simulink subsystem "battery_96_pack"  (R2022b)
settings: Solver=VariableStepAuto  StartTime=0.0  StopTime=10.0  RelTol=1e-3
values from neighbouring files (symbols this model uses):
  initial_temperature = 288.15    [battery_pack_model_data.sldd]
libraries: fl_lib x3, nesl_utility x1
settings Model: Creator=tshintai  LastModifiedBy=tshintai
settings ModelReferenceCC: EnableRefExpFcnMdlSchedulingChecks=on

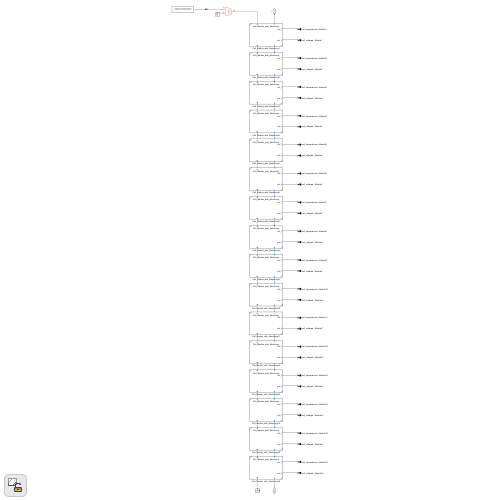
[thumbnail: Simulink's stored preview of the top-level diagram]
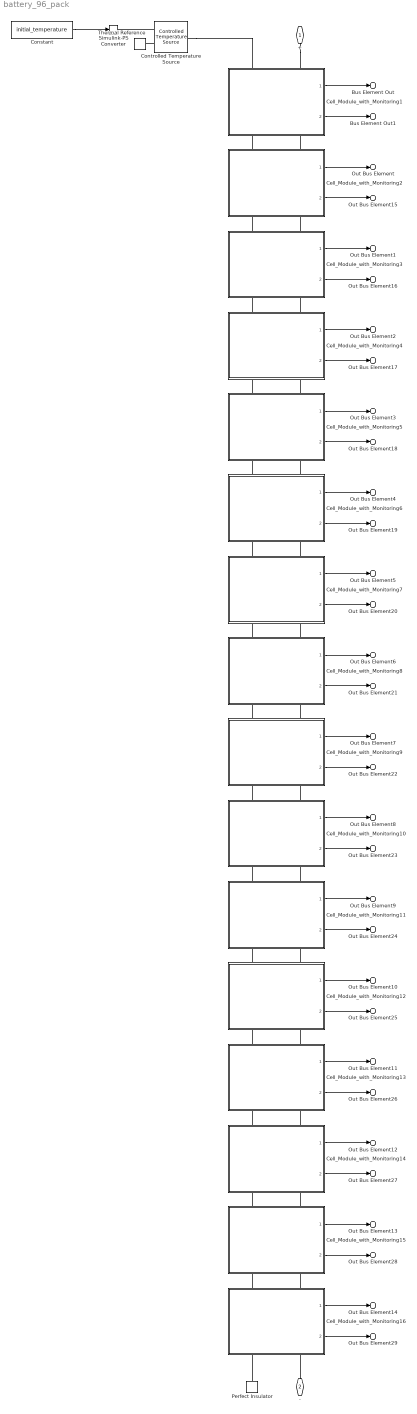
== system battery_96_pack ==
  Cell_Module_with_Monitoring{1..16} (16 alike) : Subsystem  ReferencedSubsystem=Cell_Module_with_Monitoring
      settings: PortSchema="{\"entries\":[{\"content\":{\"sides\":[{\"content\":{\"connectorIds\":[]},\"type\":\"ConnectorPlacement.EquallySpacedRectSide\",\"uuid\":\"dcef24a5-8142-4849-86b9-b18f022ccde6\"},{\"content\":{\"connectorIds\":[\"Out1\",\"Out2\"],\"side\":\"RIGHT\"},\"type\":\"ConnectorPlacement.EquallySpacedRectSide\",\"uuid\":\"d6f70724-8f5a-4fbe-99a3-1d7744c6c20b\"},{\"content\":{\"connectorIds\":[\"LConn2\",\"LConn1\"],\"side\":\"TOP\"},\"type\":\"ConnectorPlacement.EquallySpacedRectSide\",\"uuid\":\"1a464afb-99ff-42a4-8ba4-5eff5af9414c\"},{\"content\":{\"connectorIds\":[\"RConn2\",\"RConn1\"],\"side\":\"BOTTOM\"},\"type\":\"ConnectorPlacement.EquallySpacedRectSide\",\"uuid\":\"74a9329d-ffaf-4bfc-bec3-31f00c72c9b7\"}]},\"type\":\"ConnectorPlacement.EquallySpacedConnector\",\"uuid\":\"3b26f8a7-d97e-4bd5-81c6-74f00c6fb23d\"}],\"packageUris\":[\"http://schema.mathworks.com/mf0/Connector/R2020b\"],\"version\":\"1.0\"}"
  Constant : Constant  Value=initial_temperature
  Controlled Temperature Source : fl_lib/Thermal/Thermal Sources/Controlled Temperature Source
  Perfect Insulator : fl_lib/Thermal/Thermal Elements/Perfect Insulator  T_specify=off  T_priority=None  T=0 K  T_nominal_specify=off  T_nominal_unit=K  T_nominal_value=1
  Simulink-PS Converter : nesl_utility/Simulink-PS Converter  PhysicalDomain=network_engine_domain  SubClassName=ps_input  LeftPortType=input  RightPortType=output  PseudoPeriodic=off  Frequencies=[]  NoiseDistribution=none  NoiseParameters=[]  Unit=K  AffineConversion=on  FilteringAndDerivatives=provide  SimscapeFilterOrder=1  InputFilterTimeConstant=0.001  UdotUserProvided=0
  Thermal Reference : fl_lib/Thermal/Thermal Elements/Thermal Reference
  + : PMIOPort  Side=Left
  - : PMIOPort  Port=2  Side=Right
  Bus Element Out : Outport  PortName=cell_temperatures  Element=Module1
  Out Bus Element : Outport  PortName=cell_temperatures  Element=Module2
  Out Bus Element1 : Outport  PortName=cell_temperatures  Element=Module3
  Out Bus Element2 : Outport  PortName=cell_temperatures  Element=Module4
  Out Bus Element3 : Outport  PortName=cell_temperatures  Element=Module5
  Out Bus Element4 : Outport  PortName=cell_temperatures  Element=Module6
  Out Bus Element5 : Outport  PortName=cell_temperatures  Element=Module7
  Out Bus Element6 : Outport  PortName=cell_temperatures  Element=Module8
  Out Bus Element7 : Outport  PortName=cell_temperatures  Element=Module9
  Out Bus Element8 : Outport  PortName=cell_temperatures  Element=Module10
  Out Bus Element9 : Outport  PortName=cell_temperatures  Element=Module11
  Out Bus Element10 : Outport  PortName=cell_temperatures  Element=Module12
  Out Bus Element11 : Outport  PortName=cell_temperatures  Element=Module13
  Out Bus Element12 : Outport  PortName=cell_temperatures  Element=Module14
  Out Bus Element13 : Outport  PortName=cell_temperatures  Element=Module15
  Out Bus Element14 : Outport  PortName=cell_temperatures  Element=Module16
  Bus Element Out1 : Outport  Port=2  PortName=cell_voltages  Element=Module1
  Out Bus Element15 : Outport  Port=2  PortName=cell_voltages  Element=Module2
  Out Bus Element16 : Outport  Port=2  PortName=cell_voltages  Element=Module3
  Out Bus Element17 : Outport  Port=2  PortName=cell_voltages  Element=Module4
  Out Bus Element18 : Outport  Port=2  PortName=cell_voltages  Element=Module5
  Out Bus Element19 : Outport  Port=2  PortName=cell_voltages  Element=Module6
  Out Bus Element20 : Outport  Port=2  PortName=cell_voltages  Element=Module7
  Out Bus Element21 : Outport  Port=2  PortName=cell_voltages  Element=Module8
  Out Bus Element22 : Outport  Port=2  PortName=cell_voltages  Element=Module9
  Out Bus Element23 : Outport  Port=2  PortName=cell_voltages  Element=Module10
  Out Bus Element24 : Outport  Port=2  PortName=cell_voltages  Element=Module11
  Out Bus Element25 : Outport  Port=2  PortName=cell_voltages  Element=Module12
  Out Bus Element26 : Outport  Port=2  PortName=cell_voltages  Element=Module13
  Out Bus Element27 : Outport  Port=2  PortName=cell_voltages  Element=Module14
  Out Bus Element28 : Outport  Port=2  PortName=cell_voltages  Element=Module15
  Out Bus Element29 : Outport  Port=2  PortName=cell_voltages  Element=Module16
  wires:
  Cell_Module_with_Monitoring8/1 -> Out Bus Element6/1
  Cell_Module_with_Monitoring16/1 -> Out Bus Element14/1
  Cell_Module_with_Monitoring11/2 -> Out Bus Element24/1
  Cell_Module_with_Monitoring15/1 -> Out Bus Element13/1
  Cell_Module_with_Monitoring2/2 -> Out Bus Element15/1
  Cell_Module_with_Monitoring3/2 -> Out Bus Element16/1
  Cell_Module_with_Monitoring5/1 -> Out Bus Element3/1
  Cell_Module_with_Monitoring3/1 -> Out Bus Element1/1
  Cell_Module_with_Monitoring14/2 -> Out Bus Element27/1
  Cell_Module_with_Monitoring7/2 -> Out Bus Element20/1
  Cell_Module_with_Monitoring13/1 -> Out Bus Element11/1
  Cell_Module_with_Monitoring16/2 -> Out Bus Element29/1
  Cell_Module_with_Monitoring5/2 -> Out Bus Element18/1
  Cell_Module_with_Monitoring12/1 -> Out Bus Element10/1
  Cell_Module_with_Monitoring11/1 -> Out Bus Element9/1
  Cell_Module_with_Monitoring6/1 -> Out Bus Element4/1
  Cell_Module_with_Monitoring8/2 -> Out Bus Element21/1
  Cell_Module_with_Monitoring6/2 -> Out Bus Element19/1
  Cell_Module_with_Monitoring7/1 -> Out Bus Element5/1
  Cell_Module_with_Monitoring4/1 -> Out Bus Element2/1
  Cell_Module_with_Monitoring13/2 -> Out Bus Element26/1
  Cell_Module_with_Monitoring10/2 -> Out Bus Element23/1
  Cell_Module_with_Monitoring14/1 -> Out Bus Element12/1
  Cell_Module_with_Monitoring1/2 -> Bus Element Out1/1
  Cell_Module_with_Monitoring1/1 -> Bus Element Out/1
  Cell_Module_with_Monitoring10/1 -> Out Bus Element8/1
  Cell_Module_with_Monitoring15/2 -> Out Bus Element28/1
  Cell_Module_with_Monitoring4/2 -> Out Bus Element17/1
  Cell_Module_with_Monitoring9/1 -> Out Bus Element7/1
  Cell_Module_with_Monitoring9/2 -> Out Bus Element22/1
  Cell_Module_with_Monitoring12/2 -> Out Bus Element25/1
  Cell_Module_with_Monitoring2/1 -> Out Bus Element/1
  Constant/1 -> Simulink-PS Converter/1
  connections:
  +/RConn1 -- Cell_Module_with_Monitoring1/LConn1
  Cell_Module_with_Monitoring2/LConn1 -- Cell_Module_with_Monitoring1/RConn1
  Cell_Module_with_Monitoring2/LConn2 -- Cell_Module_with_Monitoring1/RConn2
  Controlled Temperature Source/LConn1 -- Cell_Module_with_Monitoring1/LConn2
  Thermal Reference/LConn1 -- Controlled Temperature Source/RConn2
  Controlled Temperature Source/RConn1 -- Simulink-PS Converter/RConn1
  Cell_Module_with_Monitoring3/LConn1 -- Cell_Module_with_Monitoring2/RConn1
  Cell_Module_with_Monitoring3/LConn2 -- Cell_Module_with_Monitoring2/RConn2
  Cell_Module_with_Monitoring4/LConn1 -- Cell_Module_with_Monitoring3/RConn1
  Cell_Module_with_Monitoring4/LConn2 -- Cell_Module_with_Monitoring3/RConn2
  Cell_Module_with_Monitoring8/LConn1 -- Cell_Module_with_Monitoring7/RConn1
  Cell_Module_with_Monitoring7/LConn1 -- Cell_Module_with_Monitoring6/RConn1
  Cell_Module_with_Monitoring6/LConn2 -- Cell_Module_with_Monitoring5/RConn2
  Cell_Module_with_Monitoring6/LConn1 -- Cell_Module_with_Monitoring5/RConn1
  Cell_Module_with_Monitoring7/LConn2 -- Cell_Module_with_Monitoring6/RConn2
  Cell_Module_with_Monitoring8/LConn2 -- Cell_Module_with_Monitoring7/RConn2
  Cell_Module_with_Monitoring5/LConn1 -- Cell_Module_with_Monitoring4/RConn1
  Cell_Module_with_Monitoring5/LConn2 -- Cell_Module_with_Monitoring4/RConn2
  Cell_Module_with_Monitoring13/LConn2 -- Cell_Module_with_Monitoring12/RConn2
  Cell_Module_with_Monitoring15/LConn2 -- Cell_Module_with_Monitoring14/RConn2
  Cell_Module_with_Monitoring14/LConn2 -- Cell_Module_with_Monitoring13/RConn2
  Cell_Module_with_Monitoring11/LConn2 -- Cell_Module_with_Monitoring10/RConn2
  Cell_Module_with_Monitoring12/LConn2 -- Cell_Module_with_Monitoring11/RConn2
  Cell_Module_with_Monitoring16/LConn2 -- Cell_Module_with_Monitoring15/RConn2
  Cell_Module_with_Monitoring10/LConn2 -- Cell_Module_with_Monitoring9/RConn2
  Cell_Module_with_Monitoring9/LConn1 -- Cell_Module_with_Monitoring8/RConn1
  Cell_Module_with_Monitoring9/LConn2 -- Cell_Module_with_Monitoring8/RConn2
  Cell_Module_with_Monitoring10/LConn1 -- Cell_Module_with_Monitoring9/RConn1
  Cell_Module_with_Monitoring11/LConn1 -- Cell_Module_with_Monitoring10/RConn1
  Cell_Module_with_Monitoring12/LConn1 -- Cell_Module_with_Monitoring11/RConn1
  Cell_Module_with_Monitoring13/LConn1 -- Cell_Module_with_Monitoring12/RConn1
  Cell_Module_with_Monitoring14/LConn1 -- Cell_Module_with_Monitoring13/RConn1
  Cell_Module_with_Monitoring15/LConn1 -- Cell_Module_with_Monitoring14/RConn1
  Cell_Module_with_Monitoring16/LConn1 -- Cell_Module_with_Monitoring15/RConn1
  -/RConn1 -- Cell_Module_with_Monitoring16/RConn1
  Perfect Insulator/LConn1 -- Cell_Module_with_Monitoring16/RConn2
